simulink model "HeartV11"  (R2024b)
settings: Solver=VariableStepAuto  StartTime=0.0  StopTime=10.0  RelTol=1e-3
libraries: Libs_unified x151
(part 1 of 2)
settings Model: Creator=ball907  LastModifiedBy=ball907

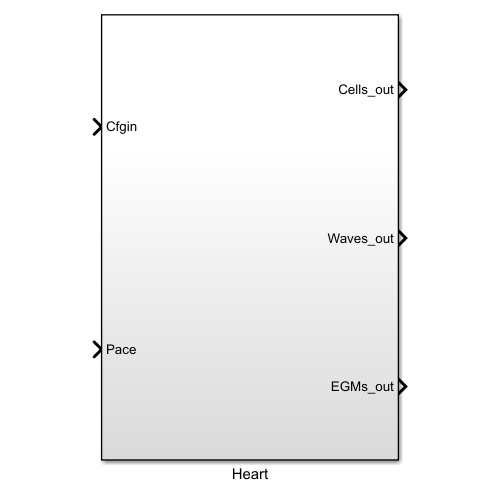
[thumbnail: Simulink's stored preview of the top-level diagram]
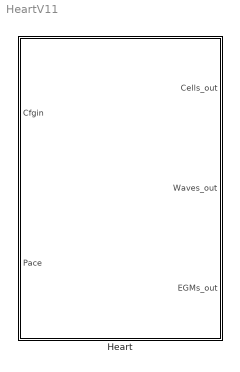
== system HeartV11 ==
  Heart : Subsystem
